simulink model "BLDC_PIL_Hall_model"  (R2026a)
settings: Solver=FixedStepDiscrete  StopTime=4  FixedStep=6.2500000000000001e-05
PostLoadFcn:
  | autombd.hsp.build.attach(bdroot);
InitFcn:
  | autombd.hsp.build.modelInitialize(bdroot);
undefined symbols (not defined in the file or in its folder): custom, motor, nxp, s32k344
libraries: BldcControllerLibrary x1, hsp_driver_lib x1
settings Model: DataDictionary=BldcData.sldd  Creator=k  LastModifiedBy=k
settings HardwareCC: ProdLargestAtomicInteger=Long  ProdLargestAtomicFloat=Double  ProdHWDeviceType=ARM Compatible->ARM Cortex-M
settings RTWCC: SystemTargetFile=autombd_s32k3.tlc  HardwareBoard=autoMBD S32K344  GenerateReport=on  Toolchain=autoMBD NXP GCC S32K344 [HSP v5-nxp_s32k3-46bb484bad882405-unconfigured]  PortableWordSizes=on  Description=autoMBD S32K3 HSP
settings STFCustomTargetCC: SystemTargetFile=autombd_s32k3.tlc  MultiwordLength=256.0  CombineOutputUpdateFcns=on  ERTCustomFileBanners=on  SupportContinuousTime=off  SupportNonInlinedSFcns=off  RemoveResetFunc=on  MATLABClassNameForMDSCustomization=Simulink.SoftwareTarget.ERTCustomization  GRTInterface=off  UseToolchainInfoCompliant=on
settings ERTTargetCC: ExtModeMexFile=noextcomm  ParMdlRefBuildCompliant=off  CompOptLevelCompliant=off  ConcurrentExecutionCompliant=off  ModelStepFunctionPrototypeControlCompliant=off  CPPClassGenCompliant=off

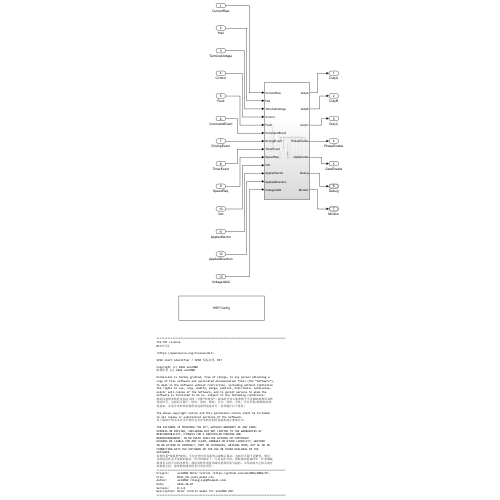
[thumbnail: Simulink's stored preview of the top-level diagram]
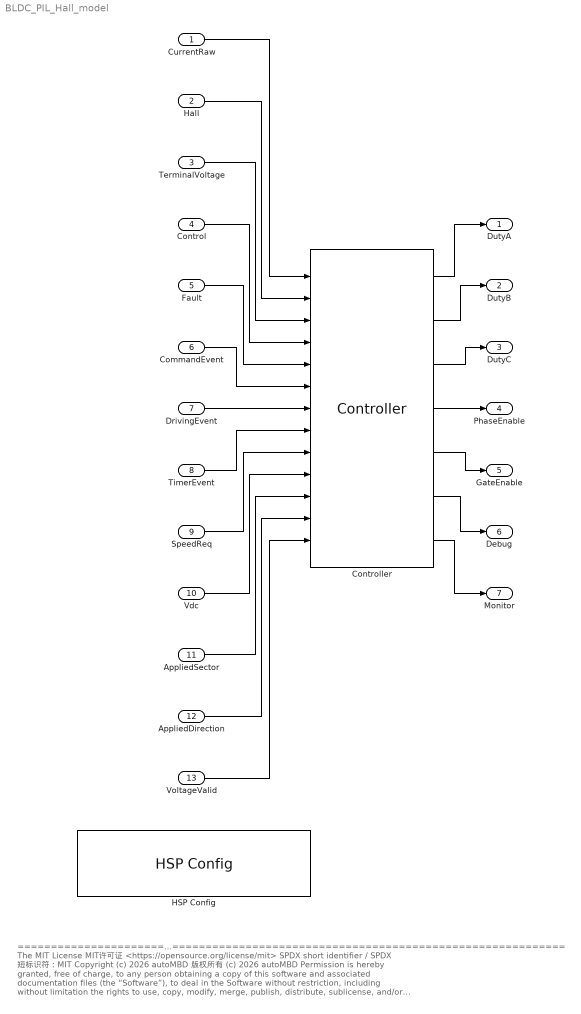
== system BLDC_PIL_Hall_model ==
  note: =================================================================================
      | The MIT License
      | MIT许可证
      |
      | <https://opensource.org/license/mit>
      |
      | SPDX short identifier / SPDX 短标识符：MIT
      |
      | Copyright (c) 2026 autoMBD
      | 版权所有 (c) 2026 autoMBD
      |
      | Permission is hereby granted, free of charge, to any person obtaining a
      | copy of this software and associated documentation files (the “Software”),
      | to deal in the Software without restriction, including without limitation
      | the rights to use, copy, modify, merge, publish, distribute, sublicense,
      | and/or sell copies of the Software, and to permit persons to whom the
      | Software is furnished to do so, subject to the following conditions:
      | 特此向获得本软件及相关文档（合称“本软件”）副本的任何人免费授予不受限制地利用本软
      | 件的许可，包括而不限于：使用、复制、修改、合并、发布、分发、分许可和/或销售本软
      | 件副本，并允许本软件的接收者也获得前述许可，但须遵守以下条件：
      |
      | The above copyright notice and this permission notice shall be included
      | in all copies or substantial portions of the Software.
      | 以上版权声明及本许可声明应包含在本软件的所有副本或主要部分中。
      |
      | THE SOFTWARE IS PROVIDED “AS IS”, WITHOUT WARRANTY OF ANY KIND,
      | EXPRESS OR IMPLIED, INCLUDING BUT NOT LIMITED TO THE WARRANTIES OF
      | MERCHANTABILITY, FITNESS FOR A PARTICULAR PURPOSE AND
      | NONINFRINGEMENT. IN NO EVENT SHALLTHE AUTHORS OR COPYRIGHT
      | HOLDERS BE LIABLE FOR ANY CLAIM, DAMAGES OR OTHER LIABILITY, WHETHER
      | IN AN ACTION OF CONTRACT, TORT OR OTHERWISE, ARISING FROM, OUT OF OR IN
      | CONNECTION WITH THE SOFTWARE OR THE USE OR OTHER DEALINGS IN THE
      | SOFTWARE.
      | 本软件系“按原样”提供，不包含任何形式的明示或默示保证，包括但不限于适销性、特定
      | 目的适用性及不侵权的保证。在任何情况下，无论是在合同、侵权或其他案件中，作者或版
      | 权持有人均不对因本软件、或因本软件的使用或其他利用而引起的、引发的或与之相关的任
      | 何权利主张、损害赔偿或其他责任承担责任。
      | =================================================================================
      | Project:     autoMBD Motor Control <https://github.com/autoMBD/AMBD-MC>
      | File:        BLDC_PIL_Hall_model.slx
      | Author:      autoMBD <tkung.lqk@foxmail.com>
      | Date:        2026-10-07
      | Version:     0.1.0
      | Description: Motor control model for autoMBD HSP.
      | =================================================================================
  CurrentRaw : Inport  OutDataTypeStr=uint16  PortDimensions=3  SampleTime=6.25e-5
  Hall : Inport  Port=2  OutDataTypeStr=uint8  PortDimensions=1  SampleTime=6.25e-5
  TerminalVoltage : Inport  Port=3  OutDataTypeStr=single  PortDimensions=3  SampleTime=6.25e-5
  Control : Inport  Port=4  OutDataTypeStr=uint8  PortDimensions=1  SampleTime=6.25e-5
  Fault : Inport  Port=5  OutDataTypeStr=boolean  PortDimensions=1  SampleTime=6.25e-5
  CommandEvent : Inport  Port=6  OutDataTypeStr=boolean  PortDimensions=1  SampleTime=6.25e-5
  DrivingEvent : Inport  Port=7  OutDataTypeStr=boolean  PortDimensions=1  SampleTime=6.25e-5
  TimerEvent : Inport  Port=8  OutDataTypeStr=boolean  PortDimensions=1  SampleTime=6.25e-5
  SpeedReq : Inport  Port=9  OutDataTypeStr=single  PortDimensions=1  SampleTime=6.25e-5
  Vdc : Inport  Port=10  OutDataTypeStr=single  PortDimensions=1  SampleTime=6.25e-5
  AppliedSector : Inport  Port=11  OutDataTypeStr=uint8  PortDimensions=1  SampleTime=6.25e-5
  AppliedDirection : Inport  Port=12  OutDataTypeStr=int8  PortDimensions=1  SampleTime=6.25e-5
  VoltageValid : Inport  Port=13  OutDataTypeStr=boolean  PortDimensions=1  SampleTime=6.25e-5
  Controller : BldcControllerLibrary/Controller  SystemSampleTime=-1  VariantActivationTime=update diagram  EmptyChoice=off  PassThrough=off  PassThroughVariantControl=(default)  EmptyChoiceVariantControl=(default)  AllowFlexibleInterface=on  Latency=0  AutoFrameSizeCalculation=off
  HSP Config : hsp_driver_lib/HSP Config  EnvironmentJson="{\"schemaVersion\":2,\"adapterId\":\"nxp.s32k3\",\"status\":\"model-configuration\",\"projectRoot\":\"\",\"matlab\":{\"executable\":\"\",\"minimumCandidateRelease\":\"R2024a\"},\"device\":{\"partNumber\":\"S32K344\",\"board\":\"custom\"},\"sdk\":{\"root\":\"\",\"version\":\"7.0.1\"},\"configurationTool\":{\"id\":\"eb.tresos\",\"templateId\":\"s32k344-motor\",\"executable\":\"\",\"guiExecutable\":\"\",\"version\":\"30.0.0\",\"arguments\":[],\"guiArguments\":[],\"workingDirectory\":\"\",\"workspaceRoot\":\"\",\"projectName\":\"Hsp_S32K344_T172\",\"projectFile\":\"\",\"kind\":\"eb\"},\"externalProjectRoot\":\"..\\\\..\\\\..\\\\..\\\\mc-models\\\\hsp\\\\config\\\\S32K344\",\"generatedCodeRoot\":\"\",\"toolchain\":{\"id\":\"nxp.gcc\",\"root\":\"\",\"makeExecutable\":\"\",\"version\":\"10.2.0 BLD1728\"},\"execution\":{\"scheduler\":\"FreeRTOS\",\"basePeriodSeconds\":6.25E-5},\"freertos\":{\"root\":\"\",\"version\":\"11.1.0\"},\"python\":{\"executable\":\"\"},\"dio\":{\"activeHigh\":true},\"pil\":{\"baudRate\":115200,\"port\":\"\",\"channelId\":-1,\"uartHandle\":\"\",\"uartInstance\":-1,\"rxPin\":\"\",\"txPin\":\"\"},\"deployment\":{\"executable\":\"\",\"provider\":\"pemicro\",\"interface\":\"USBMULTILINK\",\"debugServerExecutable\":\"\",\"gdbExecutable\":\"\",\"probeSerial\":\"\",\"targetConnected\":false},\"outputRoot\":\"\",\"runtime\":{\"taskStackWords\":4096,\"taskPriority\":2,\"schedulerMode\":\"callback-task\",\"eventCallbackName\":\"Hsp_ModelEvent\",\"eventCaptureFunction\":\"Hsp_MotorCapture\",\"eventTimeoutTicks\":2,\"eventIrqPriority\":6,\"eventIrqName\":\"\",\"eventIsrName\":\"\",\"startFunction\":\"Hsp_MotorStart\",\"stopFunction\":\"Hsp_MotorStop\",\"initializationMode\":\"auto\",\"initFunction\":\"\",\"clockSetting\":\"\",\"modeSetting\":\"\",\"sources\":[\"..\\\\..\\\\..\\\\..\\\\mc-models\\\\hsp\\\\runtime\\\\hsp_motor_board.c\"],\"includeDirectories\":[\"..\\\\..\\\\..\\\\..\\\\mc-models\\\\hsp\\\\runtime\"],\"defines\":[],\"compilerFlags\":[],\"linkerFlags\":[],\"libraries\":[],\"startupSources\":[],\"linkerScript\":\"\"},\"hspOnboarding\":{\"schemaVersion\":1,\"completed\":false,\"targetId\":\"\",\"purpose\":\"build\"},\"hspConfigMaskState\":{\"schemaVersion\":1,\"parameterNames\":[\"ConfigurationTemplate\",\"MakeExecutable\",\"SchedulerMode\",\"EventCallbackName\",\"EventCaptureFunction\",\"EventTimeoutTicks\",\"EventIrqPriority\",\"EventIrqName\",\"EventIsrName\",\"StartFunction\",\"StopFunction\",\"InitializationMode\",\"ClockSetting\",\"ModeSetting\",\"PilChannelId\",\"PilUartHandle\",\"DebugServerExecutable\",\"GdbExecutable\"]}}"  TargetId=nxp.s32k3.s32k344-custom  ConfigurationTemplate=s32k344-motor  EbProjectName=Hsp_S32K344_T172  EbProjectRoot=..\..\..\..\mc-models\hsp\config\S32K344  EbArguments=[]  EbGuiArguments=[]  SdkVersion=7.0.1  GccVersion=10.2.0 BLD1728  FreertosVersion=11.1.0  EbVersion=30.0.0  BasePeriodSeconds=6.2500000000000001e-05  TaskStackWords=4096  TaskPriority=2  SchedulerMode=callback-task  EventCallbackName=Hsp_ModelEvent  EventCaptureFunction=Hsp_MotorCapture  EventTimeoutTicks=2  EventIrqPriority=6  StartFunction=Hsp_MotorStart  StopFunction=Hsp_MotorStop  InitializationMode=auto  RuntimeSources="[\"..\\\\..\\\\..\\\\..\\\\mc-models\\\\hsp\\\\runtime\\\\hsp_motor_board.c\"]"  RuntimeIncludeDirectories="[\"..\\\\..\\\\..\\\\..\\\\mc-models\\\\hsp\\\\runtime\"]"  RuntimeDefines=[]  RuntimeCompilerFlags=[]  RuntimeLinkerFlags=[]  RuntimeLibraries=[]  StartupSources=[]  PilBaudRate=115200  PilChannelId=-1  DeploymentInterface=USBMULTILINK  TargetConnected=off  BuildAction=Build  OutputDirectory=build\BLDC_PIL_Hall_model
      settings: SourceProductName=autoMBD HSP
  DutyA : Outport  OutDataTypeStr=uint16  PortDimensions=1
  DutyB : Outport  Port=2  OutDataTypeStr=uint16  PortDimensions=1
  DutyC : Outport  Port=3  OutDataTypeStr=uint16  PortDimensions=1
  PhaseEnable : Outport  Port=4  OutDataTypeStr=boolean  PortDimensions=3
  GateEnable : Outport  Port=5  OutDataTypeStr=boolean  PortDimensions=1
  Debug : Outport  Port=6  OutDataTypeStr=Bus: tBldcDebug  PortDimensions=1
  Monitor : Outport  Port=7  OutDataTypeStr=Bus: tBldcMonitor  PortDimensions=1
  wires:
  CurrentRaw/1 -> Controller/1
  Hall/1 -> Controller/2
  TerminalVoltage/1 -> Controller/3
  Control/1 -> Controller/4
  Fault/1 -> Controller/5
  CommandEvent/1 -> Controller/6
  DrivingEvent/1 -> Controller/7
  TimerEvent/1 -> Controller/8
  SpeedReq/1 -> Controller/9
  Vdc/1 -> Controller/10
  AppliedSector/1 -> Controller/11
  AppliedDirection/1 -> Controller/12
  VoltageValid/1 -> Controller/13
  Controller/1 -> DutyA/1
  Controller/2 -> DutyB/1
  Controller/3 -> DutyC/1
  Controller/4 -> PhaseEnable/1
  Controller/5 -> GateEnable/1
  Controller/6 -> Debug/1
  Controller/7 -> Monitor/1
